simulink model "MVDR_example_hdl_4x4_systolic"  (R2020a)
settings: Solver=FixedStepDiscrete  StartTime=0.0  StopTime=stoptime  RelTol=1e-3
InitFcn:
  | model_init
values from neighbouring files (symbols this model uses):
  BackSubstitutePrototype = fi(0, matrixdivbacksub_dt)    [model_init.m]
  matrixDivDelay = NumberOfCORDICIterations*10 + 86    [model_init.m]
  movavg_bitshift = nextpow2(sqrt(windowSize))    [model_init.m]
  mvdrPipelineDelay = covMatDelay+movAvgDelay+matrixDivDelay+normResponseDelay    [model_init.m]
  numArrayElements = 4    [model_init.m]
  NumberOfCORDICIterations = matrixdivin_dt.WordLength - 1    [model_init.m]
  srcAngles = [20 60]    [model_init.m]
  sv = step(steeringVector,fc,[scanAngle; 0])    [model_init.m]
  Ts = 1/fs    (= 7.8125e-09)    [model_init.m]
  windowSize = 1024    [model_init.m]
libraries: hdlsllib x249, simulink x44, commfilt2 x4, commrfcorlib x3, commsync2 x3, commrflib2 x2, commrandsrc3 x2, phasedtxrxlib x2, commdigbbndcpm2 x1, dspsolvers x1, embreciprocals x1, commdigbbndpm3 x1
(part 11 of 11)

== matlab function MVDR_example_hdl_4x4_systolic/MVDR HDL/Compute Weight Vector/Matrix Left Divide/CORDIC/4x4 Complex CORDIC Matrix Left Divide/Back Substitute 4x4 Complex CORDIC/Invert first element - Folded/CORDIC Reciprocal Normalized, Folded/Normalizer/normalizer_block ==
  data: u input; u_normalized output; is_negative output boolean size=1; shift_amount output
function [u_normalized, is_negative, shift_amount] = normalizer_block(u)
    
    [u_normalized, is_negative, shift_amount] = normalizer(u);
    
end

function [u_normalized, is_negative, shift_amount] = normalizer(u_in)
    [u_normalized_prototype, is_negative_prototype, shift_amount_prototype] = scalar_normalizer(u_in(1));
    
    u_normalized = zeros(size(u_in),'like',u_normalized_prototype);
    is_negative = zeros(size(u_in),'like',is_negative_prototype);
    shift_amount = zeros(size(u_in),'like',shift_amount_prototype);
    
    u_normalized(1) = u_normalized_prototype;
    is_negative(1) = is_negative_prototype;
    shift_amount(1) = shift_amount_prototype;
    for k = 2:numel(u_in)
        [u_normalized(k), is_negative(k), shift_amount(k)] = ...
            scalar_normalizer(u_in(k));
    end
end
    
function [u_normalized, is_negative, shift_amount] = scalar_normalizer(u_in)
    % Only works on scalars.
    [u,is_negative] = make_positive_unsigned_real(u_in);
    [u_normalized_unsigned, shift_amount_unnormalized] = normalize_unsigned(u);
    u_normalized = cast_back_to_signed(u_normalized_unsigned,u_in);
    shift_amount = normalized_shift_value(shift_amount_unnormalized,u_in);
end

function [u_normalized, shift_amount] = normalize_unsigned(u)
    
    if isfi(u) && isfixed(u)
        
        % Define constants
        shift_amount_wordlength = coder.const(ceil(log2(u.WordLength)));
        shift_amount = fi(0,0,shift_amount_wordlength,0);
        % Puff u to next power of two wordlength so binary search will work
        puffed_wordlength = coder.const(2^shift_amount_wordlength);
        myslice = coder.const(make_slice(puffed_wordlength));
        mask = coder.const(normalizer_mask(...
            puffed_wordlength,...
            shift_amount_wordlength,...
            myslice));
        
        u_stripped = stripscaling(u);
        u_puffed = cast(u_stripped,'like',fi([],0,puffed_wordlength,0));
        u_normalized = u_puffed;
        coder.unroll();
        for k = 1:length(mask)
            if bitand(mask(k),u_normalized) == 0
                % All zeros in this slice.
                % Add the shift amount
                shift_amount = bitset(shift_amount,shift_amount_wordlength-k+1);
                % Shift up the normalized value
                u_normalized = bitsll(u_normalized,myslice(k));
            end
        end
        
        % Slice out u's original size
        u_normalized = bitsliceget(u_normalized,u_puffed.WordLength,u_puffed.WordLength-u.WordLength+1);
        u_normalized = reinterpretcast(u_normalized, numerictype(0,u_normalized.WordLength,u_normalized.WordLength-1));
        
        % Adjust shift amount for puff
        shift_amount = shift_amount - (puffed_wordlength - u.WordLength);
    elseif isfi(u) && isscaleddouble(u)
        % scaled double
        [f,e] = log2(double(real(u)));
        u_normalized = fi(2*f,0,u.WordLength,u.WordLength-1,'DataType','ScaledDouble');
        shift_amount = u.WordLength - u.FractionLength - e;
    else
        % double, single
        [f,e] = log2(double(real(u)));
        u_normalized = cast(2*f,'like',u);
        shift_amount = -e+1;
    end
end

function slice = make_slice(word_length)
    shift_amount_wordlength = ceil(log2(word_length));
    slice = fi(2.^(shift_amount_wordlength-1:-1:0).',0,shift_amount_wordlength,0,...
        'SumMode','SpecifyPrecision',...
        'SumWordLength',shift_amount_wordlength,...
        'SumFractionLength',0);
end

function mask = normalizer_mask(puffed_wordlength,shift_amount_wordlength,slice)
    % Puff u to next power of two wordlength so binary search will work
    F = fimath('RoundingMethod', 'Floor', ...
        'OverflowAction', 'Wrap', ...
        'ProductMode', 'FullPrecision', ...
        'SumMode', 'KeepLSB', ...
        'SumWordLength', puffed_wordlength, ...
        'CastBeforeSum', true);
    u_puffed = fi(0,0,puffed_wordlength,0,F);
    mask = zeros(shift_amount_wordlength,1,'like',u_puffed);
    one = cast(1,'like',mask);
    % coder.unroll is necessary to get this function to constant-fold.
    for k = coder.unroll(1:length(mask))
        mask(k) = one;
        mask(k) = bitsll(mask(k),slice(k))-one;
        mask(k) = bitsll(mask(k),sum(slice(1:k)));
    end
    mask = removefimath(mask);
end

function [y,is_negative] = make_positive_unsigned_real(x)
    if isfi(x) && isfixed(x) && ~issigned(x)
        % If the fixed-point type is unsigned, then you already know that
        % it's positive, and you don't need to cast it to an unsigned type.
        y = real(x);
        is_negative = false;
    else
        T = mytypes(x);
        if real(x(1)) < 0
            is_negative = true;
            x_intermediate = -cast(real(x),'like',T.intermediate);
            y = cast(x_intermediate,'like',T.y);
        else
            is_negative = false;
            y = cast(real(x),'like',T.y);
        end
    end
end

function T = mytypes(x)
    if isfi(x) && isscaledtype(x) && issigned(x)
        % Cast signed fixed-point types to unsigned.  The additional bit is
        % to ensure that negating the lower bound does not overflow.
        T.intermediate = fi([],1,x.WordLength+1,x.FractionLength,'DataType',x.DataType);
        T.y = fi([],0,x.WordLength+1,x.FractionLength,'DataType',x.DataType);
    else
        % All other types remain the same.  Do not propagate complexity.
        T.intermediate = cast([],'like',real(x));
        T.y = cast([],'like',real(x));
    end
end

function s = normalized_shift_value(shift_value,reference)
    if isfi(reference) && isscaledtype(reference)
        s = int16(shift_value) - int16(reference.WordLength) + int16(reference.FractionLength);
    else
        s = int16(shift_value);
    end
end

function x = cast_back_to_signed(xunsigned_normalized,u_in)
    
    if isfi(xunsigned_normalized) && ...
            isscaledtype(xunsigned_normalized) && ...
            issigned(u_in)
        
        w = xunsigned_normalized.WordLength;
        F = fimath('RoundingMethod', 'Floor', ...
            'OverflowAction', 'Wrap', ...
            'ProductMode', 'FullPrecision', ...
            'SumMode', 'SpecifyPrecision', ...
            'SumWordLength', w, ...
            'SumFractionLength', w-2, ...
            'CastBeforeSum', true);
        T.xn = fi([],0,w,w-1,F,'DataType',xunsigned_normalized.DataType);
        T.x = fi([],1,w,w-2,F,'DataType',xunsigned_normalized.DataType);
        xn = reinterpretcast(xunsigned_normalized,T.xn.numerictype);
        x = cast(xn,'like',T.x);
    else
        x = xunsigned_normalized;
    end
end

== matlab function MVDR_example_hdl_4x4_systolic/MVDR HDL/Compute Weight Vector/Matrix Left Divide/CORDIC/4x4 Complex CORDIC Matrix Left Divide/Q'B, R 4x4 Complex CORDIC Systolic Array/Leading Complex Row Rotation - 2/Rotate first element to real - 1/QR 3rd and 4th Quadrant Compensation ==
  settings: fimath=fimath('RoundingMethod','Floor','OverflowAction','Wrap')
  data: x input; y input; u input; x_out output; y_out output; u_out output; v input; v_out output
function [x_out,y_out,u_out,v_out] = quadrant_compensation(x,y,u,v)
    
    if real(x(1))<0
        % Compensation for 3rd and 4th quadrants
        x_out = -x;
        y_out = -y;

        u_out = -u;
        v_out = -v;
        
    else
        x_out = x;
        y_out = y;
        
        u_out = u;
        v_out = v;

    end
    
end

== matlab function MVDR_example_hdl_4x4_systolic/MVDR HDL/Compute Weight Vector/Matrix Left Divide/CORDIC/4x4 Complex CORDIC Matrix Left Divide/Q'B, R 4x4 Complex CORDIC Systolic Array/Leading Complex Row Rotation - 2/y = u(2:end) ==
  settings: fimath=fimath('RoundingMethod','Floor','OverflowAction','Wrap')
  data: u input; y output
function y = shorten_by_1(u)

y = u(2:end);

== matlab function MVDR_example_hdl_4x4_systolic/MVDR HDL/Compute Weight Vector/Matrix Left Divide/CORDIC/4x4 Complex CORDIC Matrix Left Divide/Q'B, R 4x4 Complex CORDIC Systolic Array/Leading Complex Row Rotation - 3/Q'B, R Row Rotations - Complex/MATLAB Function ==
  settings: fimath=fimath('RoundingMethod','Floor','OverflowAction','Wrap')
  data: x input; y input; u input; x_out output; y_out output; u_out output; v input; iteration input size=1; v_out output
function [x_out,y_out,u_out,v_out] = cordic_qr_row_rotation(...
        x,y,u,v,...
        iteration)
    % This is one CORDIC rotation for the QR decomposition.
    % In the matrix equation A*X = B
    % x and y form R from A
    % u and v form Q'*B from B
    
    % Initialize output variables
    x_out = x;
    y_out = y;
    u_out = u;
    v_out = v;
    
    % Right shift the inputs for CORDIC rotations.
    x1 = bitsra(x, iteration);
    y1 = bitsra(y, iteration);
    u1 = bitsra(u, iteration);
    v1 = bitsra(v, iteration);
    if real(y(1)) < 0
        % Counter-clockwise rotation
        x_out(:) = x - y1;
        y_out(:) = y + x1;

        u_out(:) = u - v1;
        v_out(:) = v + u1;
    else
        % Clockwise rotation
        x_out(:) = x + y1;
        y_out(:) = y - x1;
    
        u_out(:) = u + v1;
        v_out(:) = v - u1;
    end
end

== matlab function MVDR_example_hdl_4x4_systolic/MVDR HDL/Compute Weight Vector/Matrix Left Divide/CORDIC/4x4 Complex CORDIC Matrix Left Divide/Q'B, R 4x4 Complex CORDIC Systolic Array/Leading Complex Row Rotation - 3/QR 3rd and 4th Quadrant Compensation ==
  settings: fimath=fimath('RoundingMethod','Floor','OverflowAction','Wrap')
  data: x input; y input; u input; x_out output; y_out output; u_out output; v input; v_out output
function [x_out,y_out,u_out,v_out] = quadrant_compensation(x,y,u,v)
    
    if real(x(1))<0
        % Compensation for 3rd and 4th quadrants
        x_out = -x;
        y_out = -y;

        u_out = -u;
        v_out = -v;
        
    else
        x_out = x;
        y_out = y;
        
        u_out = u;
        v_out = v;

    end
    
end

== matlab function MVDR_example_hdl_4x4_systolic/MVDR HDL/Compute Weight Vector/Matrix Left Divide/CORDIC/4x4 Complex CORDIC Matrix Left Divide/Q'B, R 4x4 Complex CORDIC Systolic Array/Leading Complex Row Rotation - 3/Rotate first element to real/Force imaginary part to exactly zero ==
  settings: fimath=fimath('RoundingMethod','Floor','OverflowAction','Wrap')
  data: u input; y output
function y = zero_first_element(u)
    y = u;
    y(1) = 0;
end

== matlab function MVDR_example_hdl_4x4_systolic/MVDR HDL/Compute Weight Vector/Matrix Left Divide/CORDIC/4x4 Complex CORDIC Matrix Left Divide/Q'B, R 4x4 Complex CORDIC Systolic Array/Leading Complex Row Rotation - 3/Rotate first element to real/Q'B, R Row Rotations - Real/MATLAB Function ==
  settings: fimath=fimath('RoundingMethod','Floor','OverflowAction','Wrap')
  data: x input; y input; u input; x_out output; y_out output; u_out output; v input; iteration input size=1; v_out output
function [x_out,y_out,u_out,v_out] = cordic_qr_row_rotation(...
        x,y,u,v,...
        iteration)
    % This is one CORDIC rotation for the QR decomposition.
    % In the matrix equation A*X = B
    % x and y form R from A
    % u and v form Q'*B from B
    
    % Initialize output variables
    x_out = x;
    y_out = y;
    u_out = u;
    v_out = v;
    
    % Right shift the inputs for CORDIC rotations.
    x1 = bitsra(x, iteration);
    y1 = bitsra(y, iteration);
    u1 = bitsra(u, iteration);
    v1 = bitsra(v, iteration);
    if real(y(1)) < 0
        % Counter-clockwise rotation
        x_out(:) = x - y1;
        y_out(:) = y + x1;

        u_out(:) = u - v1;
        v_out(:) = v + u1;
    else
        % Clockwise rotation
        x_out(:) = x + y1;
        y_out(:) = y - x1;
    
        u_out(:) = u + v1;
        v_out(:) = v - u1;
    end
end

== matlab function MVDR_example_hdl_4x4_systolic/MVDR HDL/Compute Weight Vector/Matrix Left Divide/CORDIC/4x4 Complex CORDIC Matrix Left Divide/Q'B, R 4x4 Complex CORDIC Systolic Array/Leading Complex Row Rotation - 3/Rotate first element to real/QR 3rd and 4th Quadrant Compensation ==
  settings: fimath=fimath('RoundingMethod','Floor','OverflowAction','Wrap')
  data: x input; y input; u input; x_out output; y_out output; u_out output; v input; v_out output
function [x_out,y_out,u_out,v_out] = quadrant_compensation(x,y,u,v)
    
    if real(x(1))<0
        % Compensation for 3rd and 4th quadrants
        x_out = -x;
        y_out = -y;

        u_out = -u;
        v_out = -v;
        
    else
        x_out = x;
        y_out = y;
        
        u_out = u;
        v_out = v;

    end
    
end

== matlab function MVDR_example_hdl_4x4_systolic/MVDR HDL/Compute Weight Vector/Matrix Left Divide/CORDIC/4x4 Complex CORDIC Matrix Left Divide/Q'B, R 4x4 Complex CORDIC Systolic Array/Leading Complex Row Rotation - 3/Rotate first element to real - 1/Force imaginary part to exactly zero ==
  settings: fimath=fimath('RoundingMethod','Floor','OverflowAction','Wrap')
  data: u input; y output
function y = zero_first_element(u)
    y = u;
    y(1) = 0;
end

== matlab function MVDR_example_hdl_4x4_systolic/MVDR HDL/Compute Weight Vector/Matrix Left Divide/CORDIC/4x4 Complex CORDIC Matrix Left Divide/Q'B, R 4x4 Complex CORDIC Systolic Array/Leading Complex Row Rotation - 3/Rotate first element to real - 1/Q'B, R Row Rotations - Real/MATLAB Function ==
  settings: fimath=fimath('RoundingMethod','Floor','OverflowAction','Wrap')
  data: x input; y input; u input; x_out output; y_out output; u_out output; v input; iteration input size=1; v_out output
function [x_out,y_out,u_out,v_out] = cordic_qr_row_rotation(...
        x,y,u,v,...
        iteration)
    % This is one CORDIC rotation for the QR decomposition.
    % In the matrix equation A*X = B
    % x and y form R from A
    % u and v form Q'*B from B
    
    % Initialize output variables
    x_out = x;
    y_out = y;
    u_out = u;
    v_out = v;
    
    % Right shift the inputs for CORDIC rotations.
    x1 = bitsra(x, iteration);
    y1 = bitsra(y, iteration);
    u1 = bitsra(u, iteration);
    v1 = bitsra(v, iteration);
    if real(y(1)) < 0
        % Counter-clockwise rotation
        x_out(:) = x - y1;
        y_out(:) = y + x1;

        u_out(:) = u - v1;
        v_out(:) = v + u1;
    else
        % Clockwise rotation
        x_out(:) = x + y1;
        y_out(:) = y - x1;
    
        u_out(:) = u + v1;
        v_out(:) = v - u1;
    end
end

== matlab function MVDR_example_hdl_4x4_systolic/MVDR HDL/Compute Weight Vector/Matrix Left Divide/CORDIC/4x4 Complex CORDIC Matrix Left Divide/Back Substitute 4x4 Complex CORDIC/Invert first element - Folded/y = x(n) ==
  settings: fimath=fimath('RoundingMethod','Floor','OverflowAction','Wrap')
  data: x input; y output; n parameter int32 size=1
function y = extract_element(x,n)
    y = x(n);
end

== matlab function MVDR_example_hdl_4x4_systolic/MVDR HDL/Compute Weight Vector/Matrix Left Divide/CORDIC/4x4 Complex CORDIC Matrix Left Divide/Q'B, R 4x4 Complex CORDIC Systolic Array/Leading Complex Row Rotation - 3/Rotate first element to real - 1/QR 3rd and 4th Quadrant Compensation ==
  settings: fimath=fimath('RoundingMethod','Floor','OverflowAction','Wrap')
  data: x input; y input; u input; x_out output; y_out output; u_out output; v input; v_out output
function [x_out,y_out,u_out,v_out] = quadrant_compensation(x,y,u,v)
    
    if real(x(1))<0
        % Compensation for 3rd and 4th quadrants
        x_out = -x;
        y_out = -y;

        u_out = -u;
        v_out = -v;
        
    else
        x_out = x;
        y_out = y;
        
        u_out = u;
        v_out = v;

    end
    
end

== matlab function MVDR_example_hdl_4x4_systolic/MVDR HDL/Compute Weight Vector/Matrix Left Divide/CORDIC/4x4 Complex CORDIC Matrix Left Divide/Q'B, R 4x4 Complex CORDIC Systolic Array/Leading Complex Row Rotation - 3/y = u(2:end) ==
  settings: fimath=fimath('RoundingMethod','Floor','OverflowAction','Wrap')
  data: u input; y output
function y = shorten_by_1(u)

y = u(2:end);

== matlab function MVDR_example_hdl_4x4_systolic/MVDR HDL/Compute Weight Vector/Matrix Left Divide/CORDIC/4x4 Complex CORDIC Matrix Left Divide/Q'B, R 4x4 Complex CORDIC Systolic Array/Leading Complex Row Rotation - 4/Q'B, R Row Rotations - Complex/MATLAB Function ==
  settings: fimath=fimath('RoundingMethod','Floor','OverflowAction','Wrap')
  data: x input; y input; u input; x_out output; y_out output; u_out output; v input; iteration input size=1; v_out output
function [x_out,y_out,u_out,v_out] = cordic_qr_row_rotation(...
        x,y,u,v,...
        iteration)
    % This is one CORDIC rotation for the QR decomposition.
    % In the matrix equation A*X = B
    % x and y form R from A
    % u and v form Q'*B from B
    
    % Initialize output variables
    x_out = x;
    y_out = y;
    u_out = u;
    v_out = v;
    
    % Right shift the inputs for CORDIC rotations.
    x1 = bitsra(x, iteration);
    y1 = bitsra(y, iteration);
    u1 = bitsra(u, iteration);
    v1 = bitsra(v, iteration);
    if real(y(1)) < 0
        % Counter-clockwise rotation
        x_out(:) = x - y1;
        y_out(:) = y + x1;

        u_out(:) = u - v1;
        v_out(:) = v + u1;
    else
        % Clockwise rotation
        x_out(:) = x + y1;
        y_out(:) = y - x1;
    
        u_out(:) = u + v1;
        v_out(:) = v - u1;
    end
end

== matlab function MVDR_example_hdl_4x4_systolic/MVDR HDL/Compute Weight Vector/Matrix Left Divide/CORDIC/4x4 Complex CORDIC Matrix Left Divide/Q'B, R 4x4 Complex CORDIC Systolic Array/Leading Complex Row Rotation - 4/QR 3rd and 4th Quadrant Compensation ==
  settings: fimath=fimath('RoundingMethod','Floor','OverflowAction','Wrap')
  data: x input; y input; u input; x_out output; y_out output; u_out output; v input; v_out output
function [x_out,y_out,u_out,v_out] = quadrant_compensation(x,y,u,v)
    
    if real(x(1))<0
        % Compensation for 3rd and 4th quadrants
        x_out = -x;
        y_out = -y;

        u_out = -u;
        v_out = -v;
        
    else
        x_out = x;
        y_out = y;
        
        u_out = u;
        v_out = v;

    end
    
end

== matlab function MVDR_example_hdl_4x4_systolic/MVDR HDL/Compute Weight Vector/Matrix Left Divide/CORDIC/4x4 Complex CORDIC Matrix Left Divide/Q'B, R 4x4 Complex CORDIC Systolic Array/Leading Complex Row Rotation - 4/Rotate first element to real/Force imaginary part to exactly zero ==
  settings: fimath=fimath('RoundingMethod','Floor','OverflowAction','Wrap')
  data: u input; y output
function y = zero_first_element(u)
    y = u;
    y(1) = 0;
end

== matlab function MVDR_example_hdl_4x4_systolic/MVDR HDL/Compute Weight Vector/Matrix Left Divide/CORDIC/4x4 Complex CORDIC Matrix Left Divide/Q'B, R 4x4 Complex CORDIC Systolic Array/Leading Complex Row Rotation - 4/Rotate first element to real/Q'B, R Row Rotations - Real/MATLAB Function ==
  settings: fimath=fimath('RoundingMethod','Floor','OverflowAction','Wrap')
  data: x input; y input; u input; x_out output; y_out output; u_out output; v input; iteration input size=1; v_out output
function [x_out,y_out,u_out,v_out] = cordic_qr_row_rotation(...
        x,y,u,v,...
        iteration)
    % This is one CORDIC rotation for the QR decomposition.
    % In the matrix equation A*X = B
    % x and y form R from A
    % u and v form Q'*B from B
    
    % Initialize output variables
    x_out = x;
    y_out = y;
    u_out = u;
    v_out = v;
    
    % Right shift the inputs for CORDIC rotations.
    x1 = bitsra(x, iteration);
    y1 = bitsra(y, iteration);
    u1 = bitsra(u, iteration);
    v1 = bitsra(v, iteration);
    if real(y(1)) < 0
        % Counter-clockwise rotation
        x_out(:) = x - y1;
        y_out(:) = y + x1;

        u_out(:) = u - v1;
        v_out(:) = v + u1;
    else
        % Clockwise rotation
        x_out(:) = x + y1;
        y_out(:) = y - x1;
    
        u_out(:) = u + v1;
        v_out(:) = v - u1;
    end
end

== matlab function MVDR_example_hdl_4x4_systolic/MVDR HDL/Compute Weight Vector/Matrix Left Divide/CORDIC/4x4 Complex CORDIC Matrix Left Divide/Back Substitute 4x4 Complex CORDIC/Invert first element - Folded1/CORDIC Reciprocal Normalized, Folded/CORDIC Reciprocal Rotations- Folded/CORDIC Divide Kernel ==
  settings: fimath=fimath('RoundingMethod','Floor','OverflowAction','Wrap')
  data: x_reg input size=1; y_reg input size=1; z_reg input size=1; x_out output size=1; x_in input size=1; y_out output size=1; z_out output size=1; count_is_positive input size=1; iteration input size=1
function [x_out,y_out,z_out] = cordic_reciprocal_kernel(...
        x_reg,y_reg,z_reg,...
        x_in,...
        count_is_positive,iteration)
    % Returns x = x, y = 0, z = y/x
    [T,F] = cordic_reciprocal_types(x_in);
    % Initialize output variables
    x_out = cast(x_in,'like',T.x);
    y_out = cast(0,'like',T.x);
    z_out = cast(0,'like',T.x);
    % The constant, 1, cast like z
    one = cast(1,'like',T.x);
    zero = cast(0,'like',T.x);
    
    if count_is_positive
        % The next values are the previous values from the register
        x = setfimath(x_reg,F);
        y = setfimath(y_reg,F);
        z = setfimath(z_reg,F);
        % Right shift the inputs for CORDIC rotations.
        x1 = bitsra(x, iteration);
        z1 = bitsra(one, iteration);
    else
        % The next values are the new input values, iteration 0
        x = setfimath(x_in,F);
        y = one;
        z = zero;
        % No shifts on iteration 0
        x1 = x;
        z1 = one;
    end
    
    if real(y(1)) < 0
        y_out(:) = y + x1;
        z_out(:) = z - z1;
    else
        y_out(:) = y - x1;
        z_out(:) = z + z1;
    end
end

function [T,F] = cordic_reciprocal_types(x)
    if isfi(x) && isscaledtype(x)
        w = x.WordLength;
        F = fimath('RoundingMethod', 'Floor', ...
            'OverflowAction', 'Wrap', ...
            'ProductMode', 'FullPrecision', ...
            'SumMode', 'SpecifyPrecision', ...
            'SumWordLength', w, ...
            'SumFractionLength', w-2, ...
            'CastBeforeSum', true);
        T.x = fi([],x.numerictype,F,'DataType',x.DataType);
    else
        F = fimath;
        T.x = cast([],'like',x);
    end
end

== matlab function MVDR_example_hdl_4x4_systolic/MVDR HDL/Compute Weight Vector/Matrix Left Divide/CORDIC/4x4 Complex CORDIC Matrix Left Divide/Q'B, R 4x4 Complex CORDIC Systolic Array/Leading Complex Row Rotation - 4/Rotate first element to real/QR 3rd and 4th Quadrant Compensation ==
  settings: fimath=fimath('RoundingMethod','Floor','OverflowAction','Wrap')
  data: x input; y input; u input; x_out output; y_out output; u_out output; v input; v_out output
function [x_out,y_out,u_out,v_out] = quadrant_compensation(x,y,u,v)
    
    if real(x(1))<0
        % Compensation for 3rd and 4th quadrants
        x_out = -x;
        y_out = -y;

        u_out = -u;
        v_out = -v;
        
    else
        x_out = x;
        y_out = y;
        
        u_out = u;
        v_out = v;

    end
    
end

== matlab function MVDR_example_hdl_4x4_systolic/MVDR HDL/Compute Weight Vector/Matrix Left Divide/CORDIC/4x4 Complex CORDIC Matrix Left Divide/Q'B, R 4x4 Complex CORDIC Systolic Array/Leading Complex Row Rotation - 4/Rotate first element to real - 1/Force imaginary part to exactly zero ==
  settings: fimath=fimath('RoundingMethod','Floor','OverflowAction','Wrap')
  data: u input; y output
function y = zero_first_element(u)
    y = u;
    y(1) = 0;
end

== matlab function MVDR_example_hdl_4x4_systolic/MVDR HDL/Compute Weight Vector/Matrix Left Divide/CORDIC/4x4 Complex CORDIC Matrix Left Divide/Q'B, R 4x4 Complex CORDIC Systolic Array/Leading Complex Row Rotation - 4/Rotate first element to real - 1/Q'B, R Row Rotations - Real/MATLAB Function ==
  settings: fimath=fimath('RoundingMethod','Floor','OverflowAction','Wrap')
  data: x input; y input; u input; x_out output; y_out output; u_out output; v input; iteration input size=1; v_out output
function [x_out,y_out,u_out,v_out] = cordic_qr_row_rotation(...
        x,y,u,v,...
        iteration)
    % This is one CORDIC rotation for the QR decomposition.
    % In the matrix equation A*X = B
    % x and y form R from A
    % u and v form Q'*B from B
    
    % Initialize output variables
    x_out = x;
    y_out = y;
    u_out = u;
    v_out = v;
    
    % Right shift the inputs for CORDIC rotations.
    x1 = bitsra(x, iteration);
    y1 = bitsra(y, iteration);
    u1 = bitsra(u, iteration);
    v1 = bitsra(v, iteration);
    if real(y(1)) < 0
        % Counter-clockwise rotation
        x_out(:) = x - y1;
        y_out(:) = y + x1;

        u_out(:) = u - v1;
        v_out(:) = v + u1;
    else
        % Clockwise rotation
        x_out(:) = x + y1;
        y_out(:) = y - x1;
    
        u_out(:) = u + v1;
        v_out(:) = v - u1;
    end
end

== matlab function MVDR_example_hdl_4x4_systolic/MVDR HDL/Compute Weight Vector/Matrix Left Divide/CORDIC/4x4 Complex CORDIC Matrix Left Divide/Q'B, R 4x4 Complex CORDIC Systolic Array/Leading Complex Row Rotation - 4/Rotate first element to real - 1/QR 3rd and 4th Quadrant Compensation ==
  settings: fimath=fimath('RoundingMethod','Floor','OverflowAction','Wrap')
  data: x input; y input; u input; x_out output; y_out output; u_out output; v input; v_out output
function [x_out,y_out,u_out,v_out] = quadrant_compensation(x,y,u,v)
    
    if real(x(1))<0
        % Compensation for 3rd and 4th quadrants
        x_out = -x;
        y_out = -y;

        u_out = -u;
        v_out = -v;
        
    else
        x_out = x;
        y_out = y;
        
        u_out = u;
        v_out = v;

    end
    
end

== matlab function MVDR_example_hdl_4x4_systolic/MVDR HDL/Compute Weight Vector/Matrix Left Divide/CORDIC/4x4 Complex CORDIC Matrix Left Divide/Q'B, R 4x4 Complex CORDIC Systolic Array/Leading Complex Row Rotation - 4/y = u(2:end) ==
  settings: fimath=fimath('RoundingMethod','Floor','OverflowAction','Wrap')
  data: u input; y output
function y = shorten_by_1(u)

y = u(2:end);

== matlab function MVDR_example_hdl_4x4_systolic/MVDR HDL/Compute Weight Vector/Matrix Left Divide/CORDIC/4x4 Complex CORDIC Matrix Left Divide/Q'B, R 4x4 Complex CORDIC Systolic Array/Rotate first element to real/Force imaginary part to exactly zero ==
  settings: fimath=fimath('RoundingMethod','Floor','OverflowAction','Wrap')
  data: u input; y output
function y = zero_first_element(u)
    y = u;
    y(1) = 0;
end

== matlab function MVDR_example_hdl_4x4_systolic/MVDR HDL/Compute Weight Vector/Matrix Left Divide/CORDIC/4x4 Complex CORDIC Matrix Left Divide/Q'B, R 4x4 Complex CORDIC Systolic Array/Rotate first element to real/Q'B, R Row Rotations - Real/MATLAB Function ==
  settings: fimath=fimath('RoundingMethod','Floor','OverflowAction','Wrap')
  data: x input; y input; u input; x_out output; y_out output; u_out output; v input; iteration input size=1; v_out output
function [x_out,y_out,u_out,v_out] = cordic_qr_row_rotation(...
        x,y,u,v,...
        iteration)
    % This is one CORDIC rotation for the QR decomposition.
    % In the matrix equation A*X = B
    % x and y form R from A
    % u and v form Q'*B from B
    
    % Initialize output variables
    x_out = x;
    y_out = y;
    u_out = u;
    v_out = v;
    
    % Right shift the inputs for CORDIC rotations.
    x1 = bitsra(x, iteration);
    y1 = bitsra(y, iteration);
    u1 = bitsra(u, iteration);
    v1 = bitsra(v, iteration);
    if real(y(1)) < 0
        % Counter-clockwise rotation
        x_out(:) = x - y1;
        y_out(:) = y + x1;

        u_out(:) = u - v1;
        v_out(:) = v + u1;
    else
        % Clockwise rotation
        x_out(:) = x + y1;
        y_out(:) = y - x1;
    
        u_out(:) = u + v1;
        v_out(:) = v - u1;
    end
end

== matlab function MVDR_example_hdl_4x4_systolic/MVDR HDL/Compute Weight Vector/Matrix Left Divide/CORDIC/4x4 Complex CORDIC Matrix Left Divide/Q'B, R 4x4 Complex CORDIC Systolic Array/Rotate first element to real/QR 3rd and 4th Quadrant Compensation ==
  settings: fimath=fimath('RoundingMethod','Floor','OverflowAction','Wrap')
  data: x input; y input; u input; x_out output; y_out output; u_out output; v input; v_out output
function [x_out,y_out,u_out,v_out] = quadrant_compensation(x,y,u,v)
    
    if real(x(1))<0
        % Compensation for 3rd and 4th quadrants
        x_out = -x;
        y_out = -y;

        u_out = -u;
        v_out = -v;
        
    else
        x_out = x;
        y_out = y;
        
        u_out = u;
        v_out = v;

    end
    
end

== matlab function MVDR_example_hdl_4x4_systolic/MVDR HDL/Compute Weight Vector/Matrix Left Divide/CORDIC/4x4 Complex CORDIC Matrix Left Divide/Back Substitute 4x4 Complex CORDIC/Invert first element - Folded1/CORDIC Reciprocal Normalized, Folded/Change sign ==
  settings: fimath=fimath('RoundingMethod','Floor','OverflowAction','Wrap')
  data: x input; y output; is_negative input
function y = change_sign(x, is_negative)
    if is_negative
        y = -x;
    else
        y = x;
    end
end

== matlab function MVDR_example_hdl_4x4_systolic/MVDR HDL/Compute Weight Vector/Matrix Left Divide/CORDIC/4x4 Complex CORDIC Matrix Left Divide/Back Substitute 4x4 Complex CORDIC/Invert first element - Folded1/CORDIC Reciprocal Normalized, Folded/Normalizer/normalizer_block ==
  data: u input; u_normalized output; is_negative output boolean size=1; shift_amount output
function [u_normalized, is_negative, shift_amount] = normalizer_block(u)
    
    [u_normalized, is_negative, shift_amount] = normalizer(u);
    
end

function [u_normalized, is_negative, shift_amount] = normalizer(u_in)
    [u_normalized_prototype, is_negative_prototype, shift_amount_prototype] = scalar_normalizer(u_in(1));
    
    u_normalized = zeros(size(u_in),'like',u_normalized_prototype);
    is_negative = zeros(size(u_in),'like',is_negative_prototype);
    shift_amount = zeros(size(u_in),'like',shift_amount_prototype);
    
    u_normalized(1) = u_normalized_prototype;
    is_negative(1) = is_negative_prototype;
    shift_amount(1) = shift_amount_prototype;
    for k = 2:numel(u_in)
        [u_normalized(k), is_negative(k), shift_amount(k)] = ...
            scalar_normalizer(u_in(k));
    end
end
    
function [u_normalized, is_negative, shift_amount] = scalar_normalizer(u_in)
    % Only works on scalars.
    [u,is_negative] = make_positive_unsigned_real(u_in);
    [u_normalized_unsigned, shift_amount_unnormalized] = normalize_unsigned(u);
    u_normalized = cast_back_to_signed(u_normalized_unsigned,u_in);
    shift_amount = normalized_shift_value(shift_amount_unnormalized,u_in);
end

function [u_normalized, shift_amount] = normalize_unsigned(u)
    
    if isfi(u) && isfixed(u)
        
        % Define constants
        shift_amount_wordlength = coder.const(ceil(log2(u.WordLength)));
        shift_amount = fi(0,0,shift_amount_wordlength,0);
        % Puff u to next power of two wordlength so binary search will work
        puffed_wordlength = coder.const(2^shift_amount_wordlength);
        myslice = coder.const(make_slice(puffed_wordlength));
        mask = coder.const(normalizer_mask(...
            puffed_wordlength,...
            shift_amount_wordlength,...
            myslice));
        
        u_stripped = stripscaling(u);
        u_puffed = cast(u_stripped,'like',fi([],0,puffed_wordlength,0));
        u_normalized = u_puffed;
        coder.unroll();
        for k = 1:length(mask)
            if bitand(mask(k),u_normalized) == 0
                % All zeros in this slice.
                % Add the shift amount
                shift_amount = bitset(shift_amount,shift_amount_wordlength-k+1);
                % Shift up the normalized value
                u_normalized = bitsll(u_normalized,myslice(k));
            end
        end
        
        % Slice out u's original size
        u_normalized = bitsliceget(u_normalized,u_puffed.WordLength,u_puffed.WordLength-u.WordLength+1);
        u_normalized = reinterpretcast(u_normalized, numerictype(0,u_normalized.WordLength,u_normalized.WordLength-1));
        
        % Adjust shift amount for puff
        shift_amount = shift_amount - (puffed_wordlength - u.WordLength);
    elseif isfi(u) && isscaleddouble(u)
        % scaled double
        [f,e] = log2(double(real(u)));
        u_normalized = fi(2*f,0,u.WordLength,u.WordLength-1,'DataType','ScaledDouble');
        shift_amount = u.WordLength - u.FractionLength - e;
    else
        % double, single
        [f,e] = log2(double(real(u)));
        u_normalized = cast(2*f,'like',u);
        shift_amount = -e+1;
    end
end

function slice = make_slice(word_length)
    shift_amount_wordlength = ceil(log2(word_length));
    slice = fi(2.^(shift_amount_wordlength-1:-1:0).',0,shift_amount_wordlength,0,...
        'SumMode','SpecifyPrecision',...
        'SumWordLength',shift_amount_wordlength,...
        'SumFractionLength',0);
end

function mask = normalizer_mask(puffed_wordlength,shift_amount_wordlength,slice)
    % Puff u to next power of two wordlength so binary search will work
    F = fimath('RoundingMethod', 'Floor', ...
        'OverflowAction', 'Wrap', ...
        'ProductMode', 'FullPrecision', ...
        'SumMode', 'KeepLSB', ...
        'SumWordLength', puffed_wordlength, ...
        'CastBeforeSum', true);
    u_puffed = fi(0,0,puffed_wordlength,0,F);
    mask = zeros(shift_amount_wordlength,1,'like',u_puffed);
    one = cast(1,'like',mask);
    % coder.unroll is necessary to get this function to constant-fold.
    for k = coder.unroll(1:length(mask))
        mask(k) = one;
        mask(k) = bitsll(mask(k),slice(k))-one;
        mask(k) = bitsll(mask(k),sum(slice(1:k)));
    end
    mask = removefimath(mask);
end

function [y,is_negative] = make_positive_unsigned_real(x)
    if isfi(x) && isfixed(x) && ~issigned(x)
        % If the fixed-point type is unsigned, then you already know that
        % it's positive, and you don't need to cast it to an unsigned type.
        y = real(x);
        is_negative = false;
    else
        T = mytypes(x);
        if real(x(1)) < 0
            is_negative = true;
            x_intermediate = -cast(real(x),'like',T.intermediate);
            y = cast(x_intermediate,'like',T.y);
        else
            is_negative = false;
            y = cast(real(x),'like',T.y);
        end
    end
end

function T = mytypes(x)
    if isfi(x) && isscaledtype(x) && issigned(x)
        % Cast signed fixed-point types to unsigned.  The additional bit is
        % to ensure that negating the lower bound does not overflow.
        T.intermediate = fi([],1,x.WordLength+1,x.FractionLength,'DataType',x.DataType);
        T.y = fi([],0,x.WordLength+1,x.FractionLength,'DataType',x.DataType);
    else
        % All other types remain the same.  Do not propagate complexity.
        T.intermediate = cast([],'like',real(x));
        T.y = cast([],'like',real(x));
    end
end

function s = normalized_shift_value(shift_value,reference)
    if isfi(reference) && isscaledtype(reference)
        s = int16(shift_value) - int16(reference.WordLength) + int16(reference.FractionLength);
    else
        s = int16(shift_value);
    end
end

function x = cast_back_to_signed(xunsigned_normalized,u_in)
    
    if isfi(xunsigned_normalized) && ...
            isscaledtype(xunsigned_normalized) && ...
            issigned(u_in)
        
        w = xunsigned_normalized.WordLength;
        F = fimath('RoundingMethod', 'Floor', ...
            'OverflowAction', 'Wrap', ...
            'ProductMode', 'FullPrecision', ...
            'SumMode', 'SpecifyPrecision', ...
            'SumWordLength', w, ...
            'SumFractionLength', w-2, ...
            'CastBeforeSum', true);
        T.xn = fi([],0,w,w-1,F,'DataType',xunsigned_normalized.DataType);
        T.x = fi([],1,w,w-2,F,'DataType',xunsigned_normalized.DataType);
        xn = reinterpretcast(xunsigned_normalized,T.xn.numerictype);
        x = cast(xn,'like',T.x);
    else
        x = xunsigned_normalized;
    end
end
